simulink model "voter_logic"  (Simulink 8.7)
settings: Solver=FixedStepDiscrete  StartTime=0.0  StopTime=10.0  FixedStep=1  RelTol=1e-3
libraries: sldvlib x10, simulink x5
settings Model: Creator=E403510  LastModifiedBy=E403510
settings DataIOCC: SaveFormat=Dataset
settings DebuggingCC: UnderspecifiedInitializationDetection=Simplified  MergeDetectMultiDrivingBlocksExec=error  AllowSymbolicDim=off
settings HardwareCC: ProdBitPerPointer=64  ProdLargestAtomicFloat=Float  ProdIntDivRoundTo=Zero  ProdEndianess=LittleEndian  ProdWordSize=64  ProdHWDeviceType=Intel->x86-64 (Windows64)
settings GRTTargetCC: GeneratePreprocessorConditionals=Use local settings
settings ConfigComp: CovModelRefEnable=off

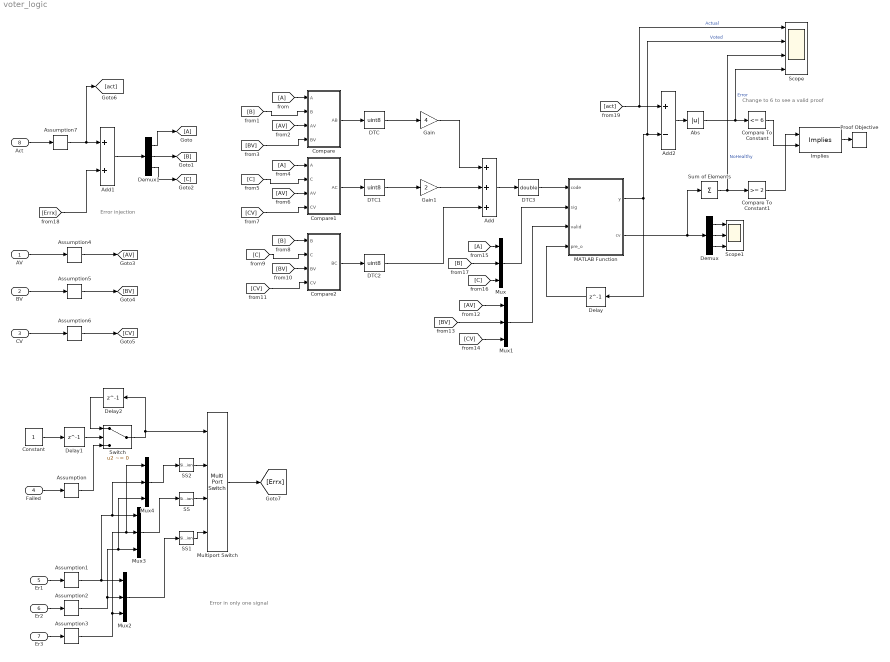
== system voter_logic ==
  note: Change to 6 to see a valid proof
  note: Error in only one signal
  note: Error injection
  AV : Inport
  BV : Inport  Port=2
  CV : Inport  Port=3
  Failed : Inport  Port=4
  Er1 : Inport  Port=5
  Er2 : Inport  Port=6
  Er3 : Inport  Port=7
  Act : Inport  Port=8
  Abs : Abs
  Add : Sum  Inputs=+++
  Add1 : Sum
  Add2 : Sum  Inputs=+-
  Assumption : sldvlib/Objectives and Constraints/Assumption  enabled=on  customAVTBlockType=Assumption  intervals={1,2,3}  initial=off  dispValues=on  outEnabled=on
      settings: AttributesFormatString=%<intervals>
  Assumption1 : sldvlib/Objectives and Constraints/Assumption  enabled=on  customAVTBlockType=Assumption  intervals={[-3 3]}  initial=off  dispValues=on  outEnabled=on
      settings: AttributesFormatString=%<intervals>
  Assumption2 : sldvlib/Objectives and Constraints/Assumption  enabled=on  customAVTBlockType=Assumption  intervals={[-3 3]}  initial=off  dispValues=on  outEnabled=on
      settings: AttributesFormatString=%<intervals>
  Assumption3 : sldvlib/Objectives and Constraints/Assumption  enabled=on  customAVTBlockType=Assumption  intervals="{[-40  40]}"  initial=off  dispValues=on  outEnabled=on
      settings: AttributesFormatString=%<intervals>
  Assumption4 : sldvlib/Objectives and Constraints/Assumption  enabled=on  customAVTBlockType=Assumption  intervals={0,1}  initial=off  dispValues=on  outEnabled=on
      settings: AttributesFormatString=%<intervals>
  Assumption5 : sldvlib/Objectives and Constraints/Assumption  enabled=on  customAVTBlockType=Assumption  intervals={0,1}  initial=off  dispValues=on  outEnabled=on
      settings: AttributesFormatString=%<intervals>
  Assumption6 : sldvlib/Objectives and Constraints/Assumption  enabled=on  customAVTBlockType=Assumption  intervals={0,1}  initial=off  dispValues=on  outEnabled=on
      settings: AttributesFormatString=%<intervals>
  Assumption7 : sldvlib/Objectives and Constraints/Assumption  enabled=on  customAVTBlockType=Assumption  intervals={[60 300]}  initial=off  dispValues=on  outEnabled=on
      settings: AttributesFormatString=%<intervals>
  Compare : Subsystem
  Compare To Constant : simulink/Logic and Bit Operations/Compare To Constant  relop=<=  const=6  OutDataTypeStr=boolean
  Compare To Constant1 : simulink/Logic and Bit Operations/Compare To Constant  relop=>=  const=2  OutDataTypeStr=boolean
  Compare1 : Subsystem
  Compare2 : Subsystem
  Constant : Constant
  DTC : DataTypeConversion  OutDataTypeStr=uint8
  DTC1 : DataTypeConversion  OutDataTypeStr=uint8
  DTC2 : DataTypeConversion  OutDataTypeStr=uint8
  DTC3 : DataTypeConversion  OutDataTypeStr=double
  Delay : Delay  DelayLength=1  InitialCondition=0
  Delay1 : Delay  DelayLength=1  InitialCondition=0
  Delay2 : Delay  DelayLength=1  InitialCondition=0
  Demux : Demux  Outputs=3
  Demux1 : Demux  Outputs=3
  Gain : Gain  Gain=4
  Gain1 : Gain  Gain=2
  Implies : sldvlib/Verification Utilities/Implies
  MATLAB Function : MATLAB Function  TreatAsAtomicUnit=on
  Multiport Switch : MultiPortSwitch
  Mux{,1..4} (5 alike) : Mux  Inputs=3
  Proof Objective : sldvlib/Objectives and Constraints/Proof Objective  enabled=on  customAVTBlockType=Proof Objective  intervals=true  dispValues=on  outEnabled=off  enableStopSim=off
      settings: AttributesFormatString=%<intervals>
  SS : SignalSpecification  Dimensions=3
  SS1 : SignalSpecification  Dimensions=3
  SS2 : SignalSpecification  Dimensions=3
  Scope : Scope  NumInputPorts=4
  Scope1 : Scope  NumInputPorts=3
  Sum of Elements : Sum  Inputs=+
  Switch : Switch  Criteria=u2 ~= 0
  wires:
  Compare/1(AB) -> DTC/1
  Compare1/1(AC) -> DTC1/1
  Compare2/1(BC) -> DTC2/1
  DTC/1 -> Gain/1
  DTC1/1 -> Gain1/1
  Gain/1 -> Add/1
  Gain1/1 -> Add/2
  DTC2/1 -> Add/3
  AV/1 -> Assumption4/1
  BV/1 -> Assumption5/1
  CV/1 -> Assumption6/1
  [A] -> Compare/1(A)
  [B] -> Compare/2(B)
  [AV] -> Compare/3(AV)
  [BV] -> Compare/4(BV)
  [A] -> Compare1/1(A)
  [C] -> Compare1/2(C)
  [AV] -> Compare1/3(AV)
  [CV] -> Compare1/4(CV)
  [B] -> Compare2/1(B)
  [C] -> Compare2/2(C)
  [BV] -> Compare2/3(BV)
  [CV] -> Compare2/4(CV)
  Add/1 -> DTC3/1
  Delay/1 -> MATLAB Function/4(pre_o)
  MATLAB Function/1(y) -> Scope/2, Add2/2, Delay/1  "Voted"
  Mux/1 -> MATLAB Function/2(sig)
  Mux1/1 -> MATLAB Function/3(valid)
  [AV] -> Mux1/1
  [BV] -> Mux1/2
  [CV] -> Mux1/3
  [A] -> Mux/1
  [B] -> Mux/2
  [C] -> Mux/3
  MATLAB Function/2(cv) -> Sum of Elements/1, Demux/1
  Demux1/2 -> [B]
  Demux1/1 -> [A]
  Demux1/3 -> [C]
  Add1/1 -> Demux1/1
  [Errx] -> Add1/2
  Delay1/1 -> Switch/2
  Constant/1 -> Delay1/1
  Switch/1 -> Delay2/1, Multiport Switch/1
  Failed/1 -> Assumption/1
  Assumption/1 -> Switch/3
  Er1/1 -> Assumption1/1
  Er2/1 -> Assumption2/1
  Er3/1 -> Assumption3/1
  Multiport Switch/1 -> [Errx]
  Delay2/1 -> Switch/1
  Assumption4/1 -> [AV]
  Assumption5/1 -> [BV]
  Assumption6/1 -> [CV]
  Act/1 -> Assumption7/1
  Assumption7/1 -> [act], Add1/1
  [act] -> Scope/1, Add2/1  "Actual"
  Add2/1 -> Abs/1
  Abs/1 -> Scope/4, Compare To Constant/1  "Error"
  SS/1 -> Multiport Switch/3
  SS1/1 -> Multiport Switch/4
  SS2/1 -> Multiport Switch/2
  DTC3/1 -> MATLAB Function/1(code)
  Sum of Elements/1 -> Compare To Constant1/1, Scope/3  "NoHealthy"
  Compare To Constant1/1 -> Implies/1
  Compare To Constant/1 -> Implies/2
  Implies/1 -> Proof Objective/1
  Assumption1/1 -> Mux4/2, Mux3/1, Mux2/1
  Assumption2/1 -> Mux4/3, Mux3/3, Mux2/2
  Assumption3/1 -> Mux4/1, Mux3/2, Mux2/3
  Mux2/1 -> SS1/1
  Mux3/1 -> SS/1
  Mux4/1 -> SS2/1
  Demux/1 -> Scope1/1
  Demux/2 -> Scope1/2
  Demux/3 -> Scope1/3

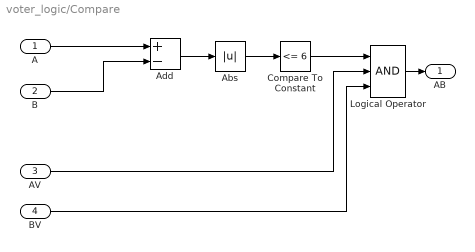
== system voter_logic/Compare ==
  A : Inport
  B : Inport  Port=2
  AV : Inport  Port=3
  BV : Inport  Port=4
  Abs : Abs
  Add : Sum  Inputs=+-
  Compare To Constant : simulink/Logic and Bit Operations/Compare To Constant  relop=<=  const=6  OutDataTypeStr=boolean
  Logical Operator : Logic  Inputs=3  AllPortsSameDT=off  OutDataTypeStr=boolean
  AB : Outport
  wires:
  Compare To Constant/1 -> Logical Operator/1
  Abs/1 -> Compare To Constant/1
  B/1 -> Add/2
  AV/1 -> Logical Operator/2
  A/1 -> Add/1
  BV/1 -> Logical Operator/3
  Add/1 -> Abs/1
  Logical Operator/1 -> AB/1

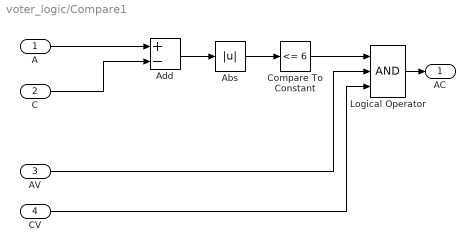
== system voter_logic/Compare1 ==
  A : Inport
  C : Inport  Port=2
  AV : Inport  Port=3
  CV : Inport  Port=4
  Abs : Abs
  Add : Sum  Inputs=+-
  Compare To Constant : simulink/Logic and Bit Operations/Compare To Constant  relop=<=  const=6  OutDataTypeStr=boolean
  Logical Operator : Logic  Inputs=3  AllPortsSameDT=off  OutDataTypeStr=boolean
  AC : Outport
  wires:
  Logical Operator/1 -> AC/1
  Add/1 -> Abs/1
  CV/1 -> Logical Operator/3
  A/1 -> Add/1
  AV/1 -> Logical Operator/2
  C/1 -> Add/2
  Abs/1 -> Compare To Constant/1
  Compare To Constant/1 -> Logical Operator/1

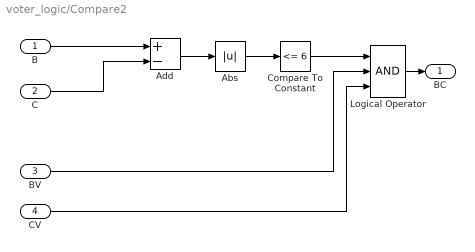
== system voter_logic/Compare2 ==
  B : Inport
  C : Inport  Port=2
  BV : Inport  Port=3
  CV : Inport  Port=4
  Abs : Abs
  Add : Sum  Inputs=+-
  Compare To Constant : simulink/Logic and Bit Operations/Compare To Constant  relop=<=  const=6  OutDataTypeStr=boolean
  Logical Operator : Logic  Inputs=3  AllPortsSameDT=off  OutDataTypeStr=boolean
  BC : Outport
  wires:
  Compare To Constant/1 -> Logical Operator/1
  Abs/1 -> Compare To Constant/1
  C/1 -> Add/2
  BV/1 -> Logical Operator/2
  B/1 -> Add/1
  CV/1 -> Logical Operator/3
  Add/1 -> Abs/1
  Logical Operator/1 -> BC/1

== matlab function MATLAB Function ==
  data: code input double; y output double; sig input double; valid input double; pre_o input double; cv output double
function [y, cv] = fcn(code,sig,valid,pre_o)
%#codegen
% AB   AC   BC  
%  0    0    0      (0) All fail
%  0    0    1      (1) A fail
%  0    1    0      (2) B fail
%  0    1    1      (3) C valid
%  1    0    0      (4) C fail
%  1    0    1      (5) B valid
%  1    1    0      (6) A valid
%  1    1    1      (7) All valid

cv = zeros(3,1);
y=0;
if code == 0
    y = pre_o;
    cv = [0;0;0];    % all fail hold prev value
elseif code == 1
    y = (sig(2)+sig(3))/2;
    cv = [0;1;1];     % A fail use average of B C
elseif code == 2
    y = (sig(1)+sig(3))/2;
    cv = [1;0;1];  % B fail use average A C
elseif code == 3
    y = sig(3);
    cv = [valid(1);valid(2);1]; % C valid
elseif code == 4
    y = (sig(1)+sig(2))/2;
    cv = [1;1;0];  % C fail use average A B
elseif code == 5
    y = sig(2);
    cv = [valid(1);1;valid(3)]; % B valid
elseif code == 6
    y = sig(1);
    cv = [1;valid(2);valid(3)]; % A valid
elseif code == 7
    y = (sig(1)+sig(2)+sig(3))/3;
    cv = [1;1;1]; % All valid
end
